simulink model "c_SCARA_2_DOF"  (R2024b)
settings: Solver=ode45  StartTime=0.0  StopTime=10  RelTol=1e-3
settings Model: Creator=Hamid Reza  LastModifiedBy=Hamid Reza
settings SolverCC: MaxConsecutiveZCs=50000

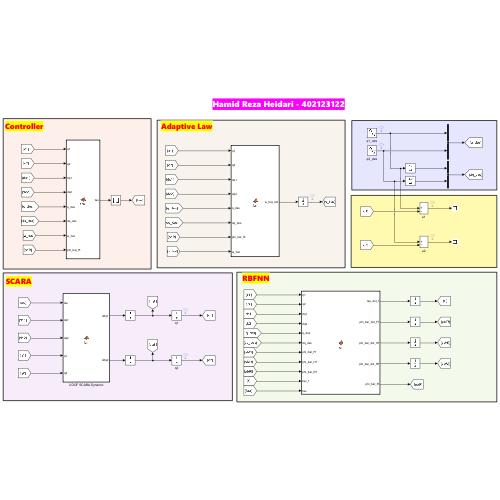
[thumbnail: Simulink's stored preview of the top-level diagram]
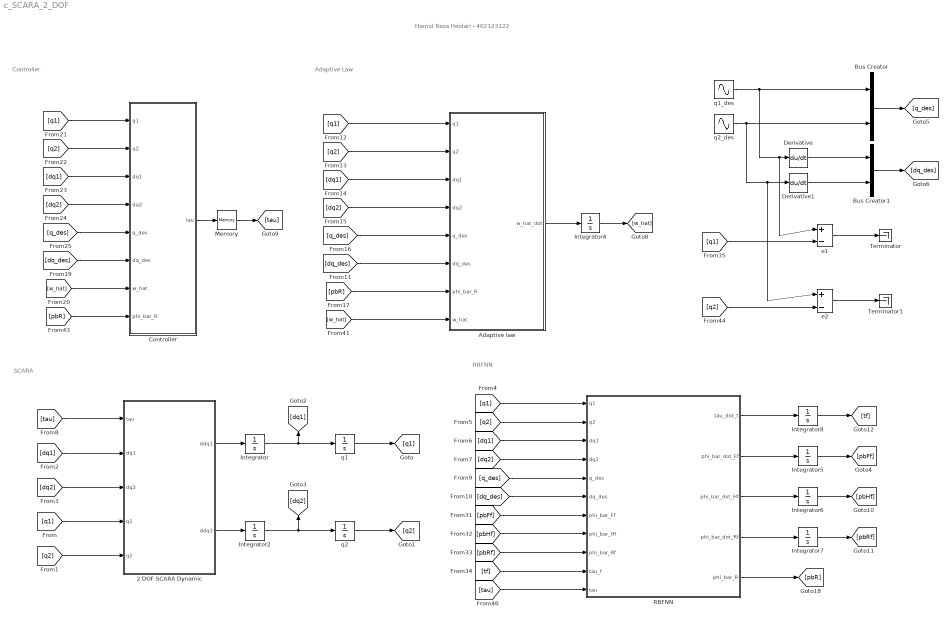
== system c_SCARA_2_DOF ==
  note: Controller
  note: RBFNN
  note: Adaptive Law
  note: SCARA
  note: Hamid Reza Heidari - 402123122
  2 DOF SCARA Dynamic : MATLAB Function  TreatAsAtomicUnit=on
  Adaptive law : MATLAB Function  TreatAsAtomicUnit=on
  Bus Creator : BusCreator  Inputs=2
  Bus Creator1 : BusCreator  Inputs=2
  Controller : MATLAB Function  TreatAsAtomicUnit=on
  Derivative : Derivative
  Derivative1 : Derivative
  Integrator : Integrator
  Integrator2 : Integrator
  Integrator4 : Integrator  InitialCondition=zeros([2 180])  ContinuousStateAttributes='w_hat'
  Integrator5 : Integrator  InitialCondition=zeros([180 1])
  Integrator6 : Integrator  InitialCondition=zeros([180 1])
  Integrator7 : Integrator  InitialCondition=zeros([180 1])
  Integrator8 : Integrator  InitialCondition=zeros([2 1])
  Memory : Memory
  RBFNN : MATLAB Function  TreatAsAtomicUnit=on
  Terminator : Terminator
  Terminator1 : Terminator
  e1 : Sum  Inputs=|+-
  e2 : Sum  Inputs=|+-
  q1 : Integrator  ContinuousStateAttributes='q1'
  q1_des : Sin  Amplitude=0.4  Frequency=0.833333  SampleTime=0
  q2 : Integrator  ContinuousStateAttributes='q2'
  q2_des : Sin  Amplitude=0.3  SampleTime=0
  wires:
  2 DOF SCARA Dynamic/1(ddq1) -> Integrator/1
  Integrator/1 -> q1/1, [dq1]
  2 DOF SCARA Dynamic/2(ddq2) -> Integrator2/1
  q1/1 -> [q1]
  q2/1 -> [q2]
  Integrator2/1 -> [dq2], q2/1
  [q2] -> 2 DOF SCARA Dynamic/5(q2)
  [q1] -> 2 DOF SCARA Dynamic/4(q1)
  [dq1] -> 2 DOF SCARA Dynamic/2(dq1)
  [dq2] -> 2 DOF SCARA Dynamic/3(dq2)
  [q1] -> RBFNN/1(q1)
  [q2] -> RBFNN/2(q2)
  [dq1] -> RBFNN/3(dq1)
  [dq2] -> RBFNN/4(dq2)
  Derivative1/1 -> Bus Creator1/2
  q2_des/1 -> Bus Creator/2, e2/1, Derivative1/1
  Derivative/1 -> Bus Creator1/1
  q1_des/1 -> e1/1, Derivative/1, Bus Creator/1
  Bus Creator/1 -> [q_des]
  Bus Creator1/1 -> [dq_des]
  [q_des] -> RBFNN/5(q_des)
  [dq_des] -> RBFNN/6(dq_des)
  [dq2] -> Adaptive law/4(dq2)
  [dq1] -> Adaptive law/3(dq1)
  [q2] -> Adaptive law/2(q2)
  [q1] -> Adaptive law/1(q1)
  [q_des] -> Adaptive law/5(q_des)
  [dq_des] -> Adaptive law/6(dq_des)
  [pbR] -> Adaptive law/7(phi_bar_R)
  Adaptive law/1(w_hat_dot) -> Integrator4/1
  Integrator4/1 -> [w_hat]
  [w_hat] -> Controller/7(w_hat)
  [dq_des] -> Controller/6(dq_des)
  [q_des] -> Controller/5(q_des)
  [dq2] -> Controller/4(dq2)
  [dq1] -> Controller/3(dq1)
  [q2] -> Controller/2(q2)
  [q1] -> Controller/1(q1)
  RBFNN/2(phi_bar_dot_Ff) -> Integrator5/1
  RBFNN/4(phi_bar_dot_Rf) -> Integrator7/1
  RBFNN/3(phi_bar_dot_Hf) -> Integrator6/1
  Integrator5/1 -> [pbFf]
  Integrator6/1 -> [pbHf]
  Integrator7/1 -> [pbRf]
  [pbRf] -> RBFNN/9(phi_bar_Rf)
  [pbHf] -> RBFNN/8(phi_bar_Hf)
  [pbFf] -> RBFNN/7(phi_bar_Ff)
  RBFNN/1(tau_dot_f) -> Integrator8/1
  Integrator8/1 -> [tf]
  [tf] -> RBFNN/10(tau_f)
  [w_hat] -> Adaptive law/8(w_hat)
  [pbR] -> Controller/8(phi_bar_R)
  RBFNN/5(phi_bar_R) -> [pbR]
  Controller/1(tau) -> Memory/1
  [q1] -> e1/2
  [q2] -> e2/2
  e1/1 -> Terminator/1
  e2/1 -> Terminator1/1
  Memory/1 -> [tau]
  [tau] -> RBFNN/11(tau)
  [tau] -> 2 DOF SCARA Dynamic/1(tau)

== matlab function c_SCARA_2_DOF/RBFNN ==
  data: q1 input; q2 input; dq1 input; dq2 input; q_des input; dq_des input; tau_dot_f output; phi_bar_Ff input; phi_bar_Hf input; phi_bar_Rf input; phi_bar_dot_Ff output; phi_bar_dot_Hf output; phi_bar_dot_Rf output; tau_f input; phi_bar_R output; tau input
function [tau_dot_f, phi_bar_dot_Ff, phi_bar_dot_Hf, phi_bar_dot_Rf, phi_bar_R] = fcn(q1, q2, dq1, dq2, q_des, dq_des, phi_bar_Ff, phi_bar_Hf, phi_bar_Rf, tau_f, tau)

N = 60;
k = 0.001;
center_range = [-2,2];
dim_z = 8;
N_center = N*3*8;

de = dq_des - [dq1;dq2];
e = q_des - [q1;q2];

N_ZERO = zeros([N 1]);

z = [q1, q2, dq1, dq2, e(1), e(2), de(1), de(2)]';

centers = linspace(center_range(1), center_range(2), N_center);

phi_F = zeros([N 1]);
phi_H = zeros([N 1]);
phi_R = zeros([N 1]);

for i = 1:1:N
    
    eta = pi;

    idx = (i-1)*(3*dim_z)+1;

    zeta_F = centers(idx:idx+dim_z-1);
    zeta_H = centers(idx+dim_z:idx+2*dim_z-1);
    zeta_R = centers(idx+2*dim_z:i+3*dim_z-1);

    phi_F(i) = phi(z, zeta_F, eta);
    phi_H(i) = phi(z, zeta_H, eta);
    phi_R(i) = phi(z, zeta_R, eta);

end

phi_bar_F = [phi_F; N_ZERO; N_ZERO];
phi_bar_H = [N_ZERO; phi_H; N_ZERO];
phi_bar_R = [N_ZERO; N_ZERO; phi_R];


phi_bar_dot_Ff = (phi_bar_F - phi_bar_Ff)/k;
phi_bar_dot_Hf = (phi_bar_H - phi_bar_Hf)/k;
phi_bar_dot_Rf = (phi_bar_R - phi_bar_Rf)/k;


tau_dot_f = ( tau - tau_f)/k;


end


function F = phi(z, zeta, eta)

F = exp((-1/eta)*norm(z-zeta)^2);

end

== matlab function c_SCARA_2_DOF/2 DOF SCARA Dynamic ==
  data: tau input; ddq1 output; ddq2 output; dq1 input; dq2 input; q1 input; q2 input
function [ddq1, ddq2] = fcn(tau, dq1, dq2, q1, q2)

m1 = 10;
m2 = 5;
l1 = 0.29;
l2 = 0.121;
g = 9.81;

m11 = (m1+m2)*l1^2 + m2*l2^2 + 2*m2*l1*l2*cos(q2);
m12 = m2*l2^2 + m2*l1*l2*cos(q2);
m21 = m12;
m22 = m2*l2^2;

M = [m11,m12;m21,m22];

c11 = -2*m2*l1*l2*dq2*sin(q2);
c12 = c11/2;
c21 = m2*l1*l2*dq1*sin(q2);
c22 = 0;

C = [c11,c12;c21,c22];

g1 = (m1+m2)*g*l1*cos(q1) + m2*g*l2*cos(q1+q2);
g2 = m2*g*l2*cos(q1+q2);

G = [g1;g2];

dq = [dq1;dq2];

ddq = inv(M)*(tau - (C*dq + G));

ddq1 = ddq(1);
ddq2 = ddq(2);

== matlab function c_SCARA_2_DOF/Controller ==
  data: q1 input; tau output; q2 input; dq1 input; dq2 input; q_des input; dq_des input; w_hat input; phi_bar_R input
function tau  = fcn(q1, q2, dq1, dq2, q_des, dq_des, w_hat, phi_bar_R)

K = [60,0;0,60];
landa = 30;

de = dq_des - [dq1;dq2];
e = q_des - [q1;q2];
s = de + landa*e;


tau = w_hat*phi_bar_R + K*s;

end

== matlab function c_SCARA_2_DOF/Adaptive law ==
  data: q1 input; q2 input; dq1 input; dq2 input; q_des input; w_hat_dot output; dq_des input; phi_bar_R input; w_hat input
function w_hat_dot = fcn(q1, q2, dq1, dq2, q_des, dq_des, phi_bar_R, w_hat)

landa = 30;
GAMMA = 10;
sigma = 0.1;
de = dq_des - [dq1;dq2];
e = q_des - [q1;q2];
s = de + landa*e;


w_hat_dot = GAMMA*(s*phi_bar_R' - sigma*w_hat);
